simulink model "BRS_Tay_compact_15b"  (R2015b)
settings: Solver=FixedStepDiscrete  StartTime=0.0  StopTime=1.0  FixedStep=1.0  RelTol=1e-3
libraries: taXlibrary x8
settings Model: Creator=emmert  LastModifiedBy=malte
settings DataIOCC: SaveFormat=Array  SignalLoggingSaveFormat=ModelDataLogs
settings OptimizationCC: ExpressionDepthLimit=2147483647
settings DebuggingCC: UnderspecifiedInitializationDetection=Classic  MergeDetectMultiDrivingBlocksExec=none  SolverPrmCheckMsg=warning  FcnCallInpInsideContextMsg=EnableAllAsWarning  AllowSymbolicDim=on  StateNameClashWarn=warning
settings HardwareCC: ProdBitPerPointer=32  ProdLargestAtomicFloat=None  ProdIntDivRoundTo=Undefined  ProdEndianess=Unspecified  ProdWordSize=32  ProdHWDeviceType=32-bit Generic
settings GRTTargetCC: GeneratePreprocessorConditionals=Disable all  CombineOutputUpdateFcns=off  GRTInterface=on
settings ConfigComp: CovModelRefEnable=Off

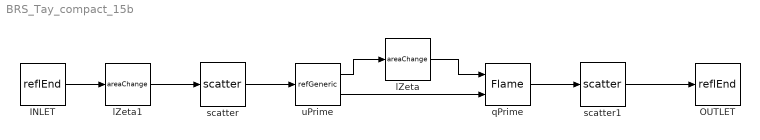
== system BRS_Tay_compact_15b ==
  INLET : taXlibrary/reflEnd  element=reflEnd  loc=Upstream  r=-0.8  A=1  Mach=0.1  rho=1.2  c=100
      settings: AttributesFormatString=%<r>
  OUTLET : taXlibrary/reflEnd  element=reflEnd  loc=Downstream  r=-0.8  A=[]  Mach=[]  rho=[]  c=[]
      settings: AttributesFormatString=%<r>
  lZeta : taXlibrary/areaChange  element=lZeta  zeta=0  lred=0  leff=0  l=1  A=4
  lZeta1 : taXlibrary/areaChange  element=lZeta  zeta=0  lred=0  leff=0  l=1  A=4
  qPrime : taXlibrary/Flame  element=rankineHugoniot  nRef=1  Mach=0.001056*101325/(287.04*293)*11.3/(101325/(287.04*1930)*0.0081*sqrt(1.4*287.04*1930))  rho=101325/(287.04*1930)  c=sqrt(1.4*287.04*1930)
  scatter : taXlibrary/scatter  element=scatteringDummy  loc=Upstream
  scatter1 : taXlibrary/scatter  element=scatteringDummy  loc=Downstream
  uPrime : taXlibrary/refGeneric  element=reference  filename=/home/thomas/tools/taX/elements/model_Luis_30kW_9.5%25.mat  modelname=model  active=off
      settings: AttributesFormatString=%<modelname>
  wires:
  lZeta/1 -> qPrime/1
  qPrime/1 -> scatter1/1
  uPrime/1 -> lZeta/1
  uPrime/2 -> qPrime/2
  scatter/1 -> uPrime/1
  lZeta1/1 -> scatter/1
  scatter1/1 -> OUTLET/1
  INLET/1 -> lZeta1/1
